simulink model "FFL"  (R2017b)
settings: Solver=VariableStepAuto  StartTime=0.0  StopTime=10.0  RelTol=1e-3
settings Model: Creator=Kalpit  LastModifiedBy=Kalpit

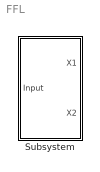
== system FFL ==
  Subsystem : Subsystem

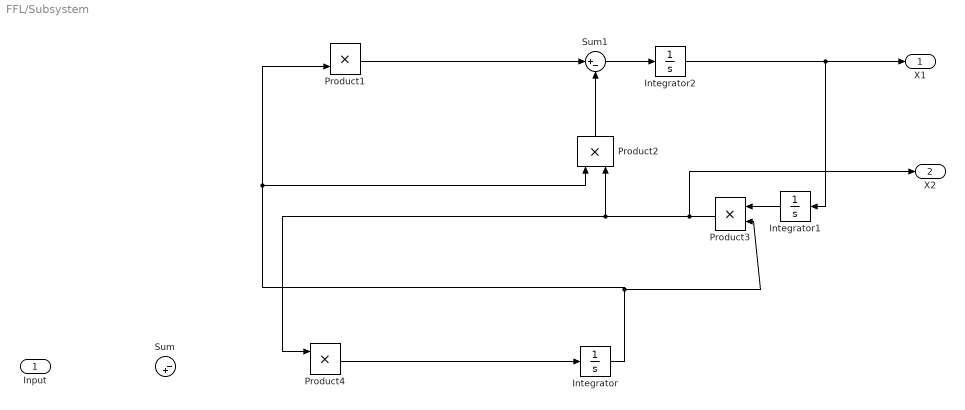
== system FFL/Subsystem ==
  Input : Inport
  Integrator : Integrator
  Integrator1 : Integrator
  Integrator2 : Integrator
  Product{1..4} (4 alike) : Product
  Sum : Sum  Inputs=|+-
  Sum1 : Sum  Inputs=|+-
  X1 : Outport
  X2 : Outport  Port=2
  wires:
  Sum1/1 -> Integrator2/1
  Product4/1 -> Integrator/1
  Integrator1/1 -> Product3/1
  Integrator2/1 -> X1/1, Integrator1/1
  Integrator/1 -> Product3/2, Product2/1, Product1/2
  Product3/1 -> X2/1, Product4/1, Product2/2
  Product1/1 -> Sum1/1
  Product2/1 -> Sum1/2
